simulink model "simpleInvertedPendulum_mdl"  (R2022b)
settings: Solver=ode4  StartTime=0.0  StopTime=1  FixedStep=.001  RelTol=1e-3
undefined symbols (not defined in the file): F, G, sys, TF
settings Model: Creator=mo780715  LastModifiedBy=mo780715

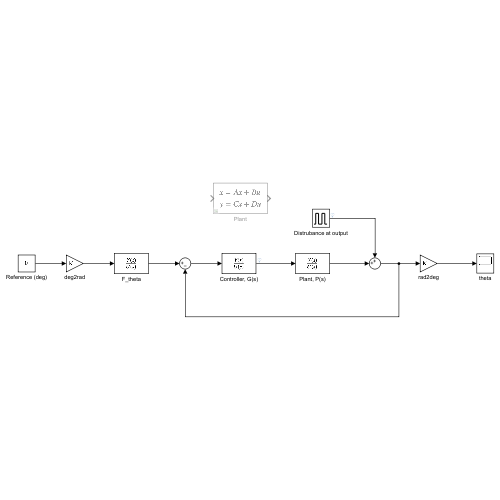
[thumbnail: Simulink's stored preview of the top-level diagram]
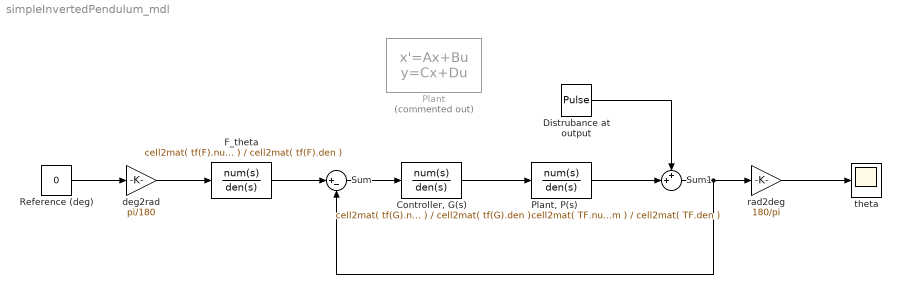
== system simpleInvertedPendulum_mdl ==
  "Controller, G(s)" : TransferFcn  Numerator=cell2mat( tf(G).num )  Denominator=cell2mat( tf(G).den )  ContinuousStateAttributes='theta'
  Distrubance at output : DiscretePulseGenerator  PulseType=Time based  Amplitude=0.1*pi/180  Period=1e6  PulseWidth=1/1e6  PhaseDelay=0.5
  F_theta : TransferFcn  Numerator=cell2mat( tf(F).num )  Denominator=cell2mat( tf(F).den )
  Plant : StateSpace  Commented=on  A=sys.A  B=sys.B  C=sys.C  D=sys.D  InitialCondition=5/180*pi  ContinuousStateAttributes='theta'
  "Plant, P(s)" : TransferFcn  Numerator=cell2mat( TF.num )  Denominator=cell2mat( TF.den )  ContinuousStateAttributes='theta'
  Reference (deg) : Constant  Value=0
  Sum : Sum  Inputs=|+-
  Sum1 : Sum  Inputs=++|
  deg2rad : Gain  Gain=pi/180
  rad2deg : Gain  Gain=180/pi
  theta : Scope
  wires:
  rad2deg/1 -> theta/1
  "Controller, G(s)"/1 -> "Plant, P(s)"/1
  Reference (deg)/1 -> deg2rad/1
  F_theta/1 -> Sum/1
  Sum/1 -> "Controller, G(s)"/1
  deg2rad/1 -> F_theta/1
  "Plant, P(s)"/1 -> Sum1/2
  Sum1/1 -> Sum/2, rad2deg/1
  Distrubance at output/1 -> Sum1/1
